simulink model "diagrama_de_olho_jitter"  (Simulink 7.7)
settings: Solver=ode3  StartTime=0.0  StopTime=1  FixedStep=2e-5  RelTol=1e-3
undefined symbols (not defined in the file): get
libraries: commsink2 x3, dsparch4 x2, commrandsrc2 x1
settings Model: Creator=Cliente  LastModifiedBy=Cliente

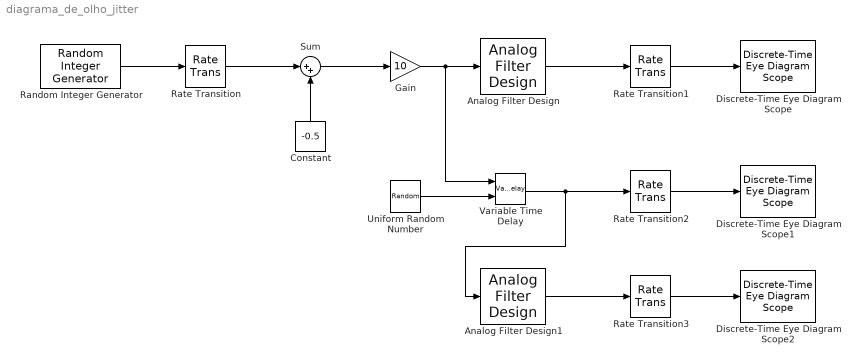
== system diagrama_de_olho_jitter ==
  Analog Filter Design : dsparch4/Analog Filter Design  method=Chebyshev I  filttype=Lowpass  N=9  Wlo=2*pi*1200  Whi=80  Rp=0.1  Rs=40
  Analog Filter Design1 : dsparch4/Analog Filter Design  method=Chebyshev I  filttype=Lowpass  N=9  Wlo=2*pi*1200  Whi=80  Rp=0.1  Rs=40
  Constant : Constant  Value=-0.5
  Discrete-Time Eye Diagram Scope : commsink2/Discrete-Time Eye Diagram Scope  Tag=EyeDiagram  SystemSampleTime=-1  sampPerSymb=50  offsetEye=0  symbPerTrace=2  numTraces=50  numNewFrames=50  LineMarkers=None  LineStyles=-  LineColors=b  dupPoints=on  fading=on  render=on  AxisGrid=on  yMin=-8  yMax=7  inphaseLabel=In-phase Amplitude  quadratureLabel=Quadrature Amplitude  openScopeAtSimStart=on  dispDiagram=In-phase and Quadrature  FrameNumber=off  FigPos=get(0,'defaultfigureposition');  figTitle=Eye Diagram  block_type_=eye  numLinesMax=8
  Discrete-Time Eye Diagram Scope1 : commsink2/Discrete-Time Eye Diagram Scope  Tag=EyeDiagram  SystemSampleTime=-1  sampPerSymb=50  offsetEye=0  symbPerTrace=2  numTraces=50  numNewFrames=50  LineMarkers=None  LineStyles=-  LineColors=b  dupPoints=on  fading=on  render=on  AxisGrid=on  yMin=-8  yMax=7  inphaseLabel=In-phase Amplitude  quadratureLabel=Quadrature Amplitude  openScopeAtSimStart=on  dispDiagram=In-phase and Quadrature  FrameNumber=off  FigPos=get(0,'defaultfigureposition');  figTitle=Eye Diagram  block_type_=eye  numLinesMax=8
  Discrete-Time Eye Diagram Scope2 : commsink2/Discrete-Time Eye Diagram Scope  Tag=EyeDiagram  SystemSampleTime=-1  sampPerSymb=50  offsetEye=0  symbPerTrace=2  numTraces=50  numNewFrames=50  LineMarkers=None  LineStyles=-  LineColors=b  dupPoints=on  fading=on  render=on  AxisGrid=on  yMin=-8  yMax=7  inphaseLabel=In-phase Amplitude  quadratureLabel=Quadrature Amplitude  openScopeAtSimStart=on  dispDiagram=In-phase and Quadrature  FrameNumber=off  FigPos=get(0,'defaultfigureposition');  figTitle=Eye Diagram  block_type_=eye  numLinesMax=8
  Gain : Gain  Gain=10
  Random Integer Generator : commrandsrc2/Random Integer Generator  SystemSampleTime=-1  mul=2  seed=randseed  Ts=1e-3  frameBased=off  sampPerFrame=1  orient=off  outDataType=double
  Rate Transition{,1..3} (4 alike) : RateTransition  OutPortSampleTime=2e-5
  Sum : Sum  Inputs=|++
  Uniform Random Number : UniformRandomNumber  Minimum=0.00002  Maximum=0.0005  SampleTime=0
  Variable Time Delay : VariableTransportDelay  MaximumDelay=0.0025  ZeroDelay=on  TransDelayFeedthrough=on
  wires:
  Random Integer Generator/1 -> Rate Transition/1
  Rate Transition/1 -> Sum/1
  Constant/1 -> Sum/2
  Sum/1 -> Gain/1
  Gain/1 -> Analog Filter Design/1, Variable Time Delay/1
  Analog Filter Design/1 -> Rate Transition1/1
  Rate Transition1/1 -> Discrete-Time Eye Diagram Scope/1
  Uniform Random Number/1 -> Variable Time Delay/2
  Variable Time Delay/1 -> Rate Transition2/1, Analog Filter Design1/1
  Analog Filter Design1/1 -> Rate Transition3/1
  Rate Transition2/1 -> Discrete-Time Eye Diagram Scope1/1
  Rate Transition3/1 -> Discrete-Time Eye Diagram Scope2/1
